simulink model "simuLinkDiagram"  (R2024a)
settings: Solver=VariableStepAuto  StartTime=0.0  StopTime=15  RelTol=1e-3
StartFcn:
  | procesamientoPorNodo=500;
  | valorReferencia=70;
  | cantidadNodos=50;
  | transaccionesEnProceso=21000;
  | porcentajeCPU=100*transaccionesEnProceso/(cantidadNodos*procesamientoPorNodo);
libraries: SignalEditorBlockLib x1
settings Model: Creator=Administrador  LastModifiedBy=SIMON
settings DataIOCC: ExternalInput=cantidadNodos

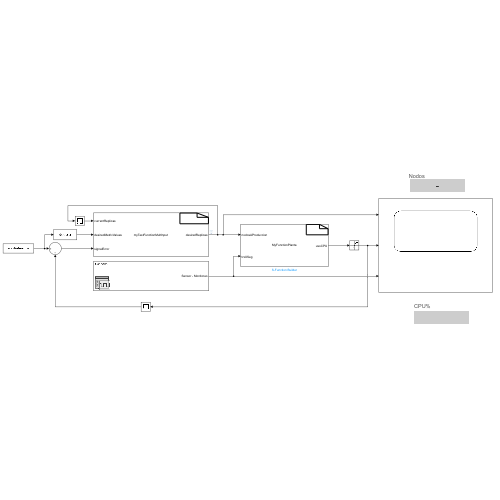
[thumbnail: Simulink's stored preview of the top-level diagram]
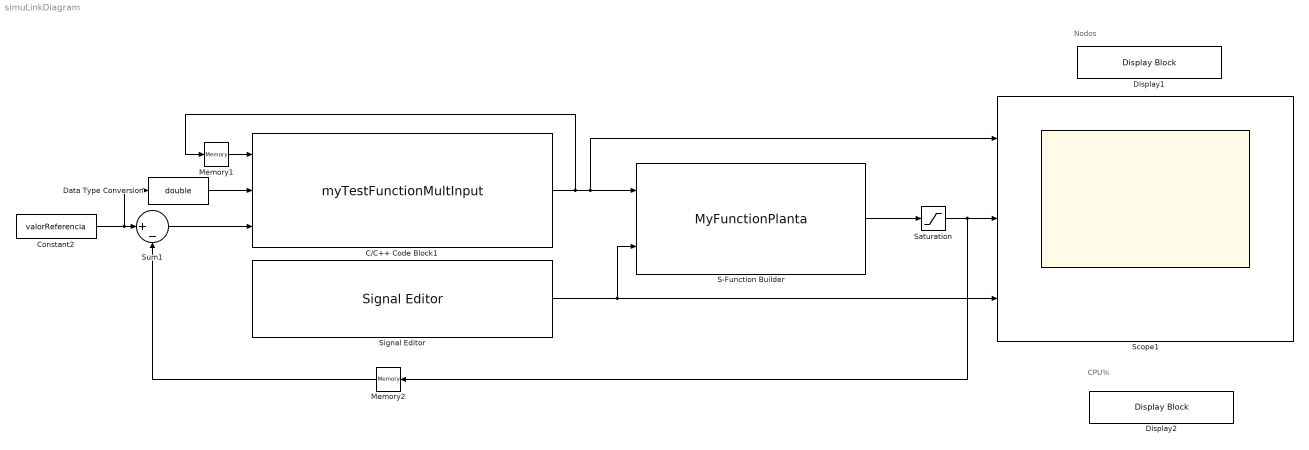
== system simuLinkDiagram ==
  note: Nodos
  note: CPU%
  C/C++ Code Block1 : S-Function  FunctionName=myTestFunctionMultInput  SFunctionModules=myTestFunctionMultInput_wrapper.c  SFunctionDeploymentMode=off  EnableBusSupport=off  mask(S-Function Builder){}
      mask help: Simulink:masks:SFunctionBuilder_MD
      mask init:
      | val = [[.9  0.75 0.75 1 1 .9 .9 1]',[1 1 0.75 0.75 .9 .9 1 .9]'];try , sys = get_param(gcb,'SfunBuilderFcnName');if isempty(sys), sys = get_param(gcb,'FunctionName'); end,catch, sys = get_param(gcb,'FunctionName'); end
      settings: CopyFcn=set_param(gcbh,'LinkStatus','none')  OpenFcn=sfunctionwizard(gcbh)
      mask Display:
      | plot(val(:,1),val(:,2))
      | disp(sys)
      | port_label('input',1,sprintf('%s', 'currentReplicas'),'interpreter','tex')
      | port_label('input',2,sprintf('%s', 'desiredMetricValues'),'interpreter','tex')
      | port_label('input',3,sprintf('%s', 'signalError'),'interpreter','tex')
      | port_label('output',1,sprintf('%s', 'desiredReplicas'),'interpreter','tex')
  Constant2 : Constant  Value=valorReferencia  OutDataTypeStr=int32
  Data Type Conversion : DataTypeConversion  OutDataTypeStr=double  SaturateOnIntegerOverflow=off  RndMeth=Floor
  Display1 : DisplayBlock  LabelPosition=Hide  Transparency=1
  Display2 : DisplayBlock  LabelPosition=Hide  Transparency=1
  Memory1 : Memory  InitialCondition=cantidadNodos  InheritSampleTime=on
  Memory2 : Memory  InheritSampleTime=on
  S-Function Builder : S-Function  FunctionName=MyFunctionPlanta  SFunctionModules=MyFunctionPlanta_wrapper.c  SFunctionDeploymentMode=off  EnableBusSupport=off  mask(S-Function Builder){}
      mask help: Simulink:masks:SFunctionBuilder_MD
      mask init: same as simuLinkDiagram/C/C++ Code Block1
      settings: CopyFcn=set_param(gcbh,'LinkStatus','none')  OpenFcn=sfunctionwizard(gcbh)
      mask Display:
      | plot(val(:,1),val(:,2))
      | disp(sys)
      | port_label('input',1,sprintf('%s', 'nodosAProduccion'),'interpreter','tex')
      | port_label('input',2,sprintf('%s', 'trxXSeg'),'interpreter','tex')
      | port_label('output',1,sprintf('%s', 'usoCPU'),'interpreter','tex')
  Saturation : Saturate  UpperLimit=100  LowerLimit=0
  Scope1 : Scope  NumInputPorts=3
  Signal Editor : SignalEditorBlockLib/Signal Editor  FileName=singal.mat  ActiveScenario=Scenario  ActiveSignal=Sensor - Monitoreo  IsBus=off  OutputBusObjectStr=Bus: BusObject  SampleTime=0  ZeroCross=off  OutputAfterFinalValue=Holding final value  Unit=inherit  PreserveSignalName=on  ApplySigPropsToAllScenarios=on  ApplySigPropsToAllSignals=off
  Sum1 : Sum  Inputs=|+-  OutDataTypeStr=double  AccumDataTypeStr=double
  wires:
  Constant2/1 -> Data Type Conversion/1, Sum1/1
  Sum1/1 -> C/C++ Code Block1/3
  C/C++ Code Block1/1 -> S-Function Builder/1, Scope1/1, Memory1/1
  Memory1/1 -> C/C++ Code Block1/1
  Signal Editor/1 -> Scope1/3, S-Function Builder/2
  S-Function Builder/1 -> Saturation/1
  Memory2/1 -> Sum1/2
  Saturation/1 -> Memory2/1, Scope1/2
  Data Type Conversion/1 -> C/C++ Code Block1/2
